simulink model "CTRL_SPECCTRL_FB_STRAT1_SLAWHL_test"  (R2024b)
settings: Solver=VariableStepAuto  StartTime=0.0  StopTime=10.0  RelTol=1e-3
libraries: CTRL_SPECCTRL_FB_STRAT1_SLAWHL x1
settings Model: Creator=blatak  LastModifiedBy=blatak

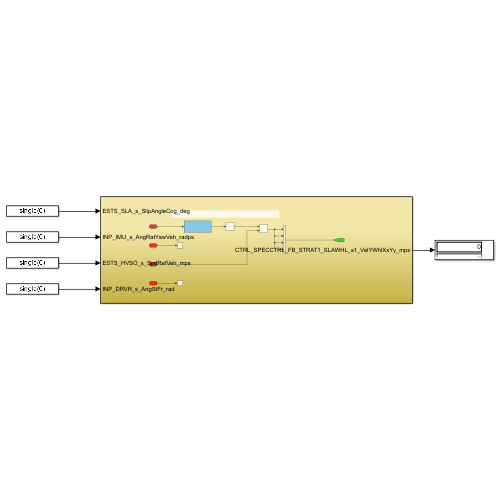
[thumbnail: Simulink's stored preview of the top-level diagram]
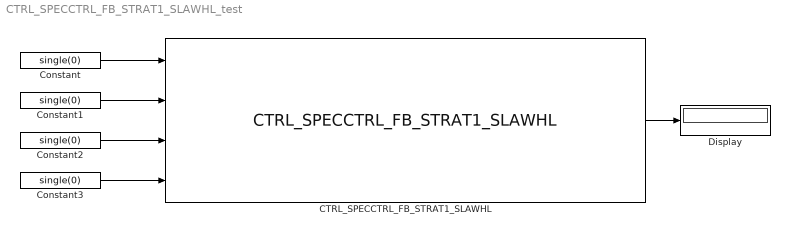
== system CTRL_SPECCTRL_FB_STRAT1_SLAWHL_test ==
  CTRL_SPECCTRL_FB_STRAT1_SLAWHL : CTRL_SPECCTRL_FB_STRAT1_SLAWHL/CTRL_SPECCTRL_FB_STRAT1_SLAWHL  SystemSampleTime=-1  VariantActivationTime=update diagram  AllowFlexibleInterface=on  Latency=0  AutoFrameSizeCalculation=off
  Constant{,1..3} (4 alike) : Constant  Value=single(0)
  Display : Display
  wires:
  Constant/1 -> CTRL_SPECCTRL_FB_STRAT1_SLAWHL/1
  Constant1/1 -> CTRL_SPECCTRL_FB_STRAT1_SLAWHL/2
  Constant3/1 -> CTRL_SPECCTRL_FB_STRAT1_SLAWHL/4
  Constant2/1 -> CTRL_SPECCTRL_FB_STRAT1_SLAWHL/3
  CTRL_SPECCTRL_FB_STRAT1_SLAWHL/1 -> Display/1
